simulink model "simula_q10"  (R2018a)
settings: Solver=VariableStepAuto  StartTime=0.0  StopTime=40  RelTol=1e-3
libraries: simulink_extras x9, simulink x6
settings Model: Creator=55479  LastModifiedBy=55479

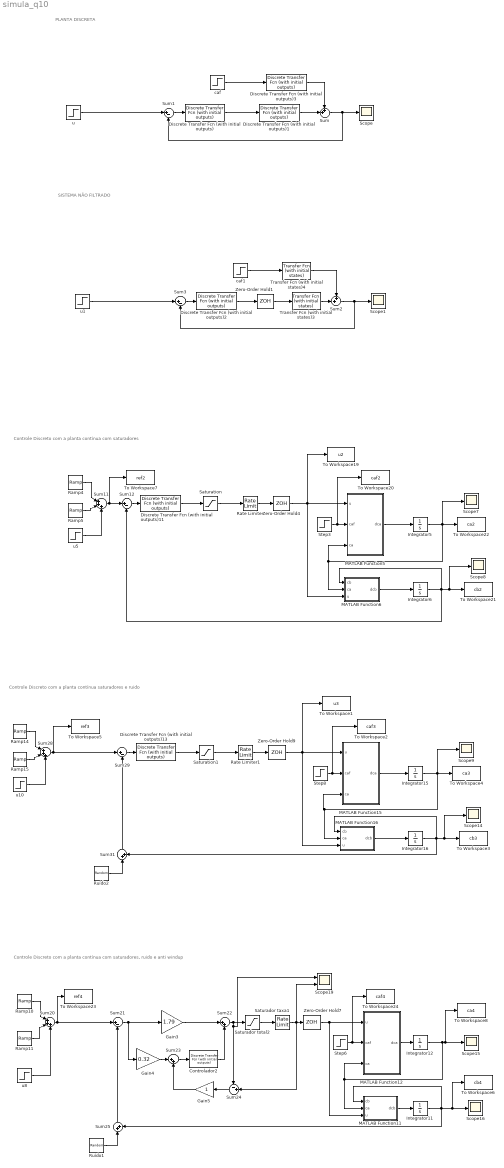
== system simula_q10 ==
  note: SISTEMA NÃO FILTRADO
  note: PLANTA DISCRETA
  note: Controle Discreto com a planta contínua com saturadores
  note: Controle Discreto com a planta contínua saturadores e ruido
  note: Controle Discreto com a planta contínua com saturadores, ruido e anti windup
  Controlador2 : simulink_extras/Additional Discrete/Discrete Transfer Fcn (with initial outputs)  N=[1 0]  D="[1  -1]"  U0=[0]  Y0=0  TS=0.08
      settings: SourceProductName=Simulink  SourceProductBaseCode=SL
  Discrete Transfer Fcn (with initial outputs) : simulink_extras/Additional Discrete/Discrete Transfer Fcn (with initial outputs)  N=[24.2704 -1.7916]  D="[1  -1]"  U0=[1]  Y0=0  TS=0.08
      settings: SourceProductName=Simulink  SourceProductBaseCode=SL
  Discrete Transfer Fcn (with initial outputs)1 : simulink_extras/Additional Discrete/Discrete Transfer Fcn (with initial outputs)  N=[0.07101]  D="[1  -0.8732]"  U0=[1]  Y0=2.345  TS=0.08
      settings: SourceProductName=Simulink  SourceProductBaseCode=SL
  Discrete Transfer Fcn (with initial outputs)11 : simulink_extras/Additional Discrete/Discrete Transfer Fcn (with initial outputs)  N=[2.11 -1.79]  D="[1  -1]"  U0=[0]  Y0=0  TS=0.08
      settings: SourceProductName=Simulink  SourceProductBaseCode=SL
  Discrete Transfer Fcn (with initial outputs)13 : simulink_extras/Additional Discrete/Discrete Transfer Fcn (with initial outputs)  N=[2.11 -1.79]  D="[1  -1]"  U0=[0]  Y0=0  TS=0.08
      settings: SourceProductName=Simulink  SourceProductBaseCode=SL
  Discrete Transfer Fcn (with initial outputs)2 : simulink_extras/Additional Discrete/Discrete Transfer Fcn (with initial outputs)  N=[4.2253 -3.585]  D="[1  -1]"  U0=[0]  Y0=0  TS=0.08
      settings: SourceProductName=Simulink  SourceProductBaseCode=SL
  Discrete Transfer Fcn (with initial outputs)3 : simulink_extras/Additional Discrete/Discrete Transfer Fcn (with initial outputs)  N=[0.05706]  D=[1 -0.8732]  U0=[0]  Y0=0  TS=0.08
      settings: SourceProductName=Simulink  SourceProductBaseCode=SL
  Gain3 : Gain  Gain=1.79
  Gain4 : Gain  Gain=0.32
  Gain5 : Gain
  Integrator{5..6,11..12,15..16} (6 alike) : Integrator
  MATLAB Function11 : MATLAB Function  TreatAsAtomicUnit=on
  MATLAB Function12 : MATLAB Function  TreatAsAtomicUnit=on
  MATLAB Function15 : MATLAB Function  TreatAsAtomicUnit=on
  MATLAB Function16 : MATLAB Function  TreatAsAtomicUnit=on
  MATLAB Function5 : MATLAB Function  TreatAsAtomicUnit=on
  MATLAB Function6 : MATLAB Function  TreatAsAtomicUnit=on
  Ramp10 : simulink/Sources/Ramp  slope=2.345/10  start=0  InitialOutput=0
  Ramp11 : simulink/Sources/Ramp  slope=-2.345/10  start=10  InitialOutput=0
  Ramp14 : simulink/Sources/Ramp  slope=2.345/10  start=0  InitialOutput=0
  Ramp15 : simulink/Sources/Ramp  slope=-2.345/10  start=10  InitialOutput=0
  Ramp4 : simulink/Sources/Ramp  slope=2.345/10  start=0  InitialOutput=0
  Ramp5 : simulink/Sources/Ramp  slope=-2.345/10  start=10  InitialOutput=0
  Rate Limiter : RateLimiter  RisingSlewLimit=2  FallingSlewLimit=-2  SampleTimeMode=inherited
  Rate Limiter1 : RateLimiter  RisingSlewLimit=2  FallingSlewLimit=-2  SampleTimeMode=inherited
  Ruído1 : RandomNumber  Variance=0.001  SampleTime=0.001
  Ruído2 : RandomNumber  Variance=0.001  SampleTime=0.001
  Saturador taxa1 : RateLimiter  RisingSlewLimit=2  FallingSlewLimit=-2  SampleTimeMode=inherited
  Saturador total2 : Saturate  UpperLimit=10  LowerLimit=0
  Saturation : Saturate  UpperLimit=10  LowerLimit=0
  Saturation1 : Saturate  UpperLimit=10  LowerLimit=0
  Scope{,1,7..9,14..16} (8 alike) : Scope
  Scope19 : Scope  NumInputPorts=2
  Step3 : Step  Time=30  Before=5.1  After=5.3  SampleTime=0
  Step6 : Step  Time=30  Before=5.1  After=5.4  SampleTime=0
  Step8 : Step  Time=30  Before=5.1  After=5.4  SampleTime=0
  Sum : Sum  Inputs=++|
  Sum{1,3,12,21,29} (5 alike) : Sum  Inputs=|+-
  Sum11 : Sum  Inputs=|+++
  Sum2 : Sum  Inputs=++|
  Sum20 : Sum  Inputs=|+++
  Sum{22..23,25,31} (4 alike) : Sum  Inputs=|++
  Sum24 : Sum  Inputs=-+|
  Sum28 : Sum  Inputs=|+++
  To Workspace1 : ToWorkspace  VariableName=u3  SaveFormat=Timeseries  SampleTime=-1
  To Workspace19 : ToWorkspace  VariableName=u2  SaveFormat=Timeseries  SampleTime=-1
  To Workspace2 : ToWorkspace  VariableName=caf3  SaveFormat=Timeseries  SampleTime=-1
  To Workspace20 : ToWorkspace  VariableName=caf2  SaveFormat=Timeseries  SampleTime=-1
  To Workspace21 : ToWorkspace  VariableName=cb2  SaveFormat=Timeseries  SampleTime=-1
  To Workspace22 : ToWorkspace  VariableName=ca2  SaveFormat=Timeseries  SampleTime=-1
  To Workspace23 : ToWorkspace  VariableName=ref4  SaveFormat=Timeseries  SampleTime=-1
  To Workspace24 : ToWorkspace  VariableName=caf4  SaveFormat=Timeseries  SampleTime=-1
  To Workspace3 : ToWorkspace  VariableName=cb3  SaveFormat=Timeseries  SampleTime=-1
  To Workspace4 : ToWorkspace  VariableName=ca3  SaveFormat=Timeseries  SampleTime=-1
  To Workspace5 : ToWorkspace  VariableName=ref3  SaveFormat=Timeseries  SampleTime=-1
  To Workspace6 : ToWorkspace  VariableName=cb4  SaveFormat=Timeseries  SampleTime=-1
  To Workspace7 : ToWorkspace  VariableName=ref2  SaveFormat=Timeseries  SampleTime=-1
  To Workspace8 : ToWorkspace  VariableName=ca4  SaveFormat=Timeseries  SampleTime=-1
  Transfer Fcn (with initial states)3 : simulink_extras/Additional Linear/Transfer Fcn (with initial states)  N=[0.56]  D=[0.59 1]  X0=0
  Transfer Fcn (with initial states)4 : simulink_extras/Additional Linear/Transfer Fcn (with initial states)  N=[0.45]  D=[0.59 1]  X0=0
  Zero-Order Hold{1,4,7,9} (4 alike) : ZeroOrderHold  SampleTime=0.08
  caf : Step  Time=10  Before=5.1  After=5.1  SampleTime=0
  caf1 : Step  Time=10  Before=5.1  After=5.1  SampleTime=0
  u : Step  Time=10  Before=2.345  After=2.545  SampleTime=0
  u1 : Step  Time=40  Before=2.345  After=2.545  SampleTime=0.08
  u10 : Step  Time=20  After=0.3  SampleTime=0
  u5 : Step  Time=20  After=0.2  SampleTime=0
  u8 : Step  Time=20  After=0.3  SampleTime=0
  wires:
  Sum/1 -> Sum1/2, Scope/1
  Sum1/1 -> Discrete Transfer Fcn (with initial outputs)/1
  caf/1 -> Discrete Transfer Fcn (with initial outputs)3/1
  u/1 -> Sum1/1
  Zero-Order Hold1/1 -> Transfer Fcn (with initial states)3/1
  Transfer Fcn (with initial states)3/1 -> Sum2/2
  Sum3/1 -> Discrete Transfer Fcn (with initial outputs)2/1
  u1/1 -> Sum3/1
  Sum2/1 -> Scope1/1, Sum3/2
  Transfer Fcn (with initial states)4/1 -> Sum2/1
  Discrete Transfer Fcn (with initial outputs)2/1 -> Zero-Order Hold1/1
  caf1/1 -> Transfer Fcn (with initial states)4/1
  Discrete Transfer Fcn (with initial outputs)3/1 -> Sum/1
  Discrete Transfer Fcn (with initial outputs)1/1 -> Sum/2
  Discrete Transfer Fcn (with initial outputs)/1 -> Discrete Transfer Fcn (with initial outputs)1/1
  Ramp5/1 -> Sum11/2
  MATLAB Function5/1(dca) -> Integrator5/1
  u5/1 -> Sum11/3
  MATLAB Function6/1(dcb) -> Integrator6/1
  Ramp4/1 -> Sum11/1
  Integrator6/1 -> Sum12/2, MATLAB Function6/1(cb), Scope8/1, To Workspace21/1
  Step3/1 -> To Workspace20/1, MATLAB Function5/2(caf)
  Sum12/1 -> Discrete Transfer Fcn (with initial outputs)11/1
  Zero-Order Hold4/1 -> To Workspace19/1, MATLAB Function6/3(u), MATLAB Function5/1(u)
  Integrator5/1 -> To Workspace22/1, Scope7/1, MATLAB Function6/2(ca), MATLAB Function5/3(ca)
  Saturation/1 -> Rate Limiter/1
  Rate Limiter/1 -> Zero-Order Hold4/1
  Discrete Transfer Fcn (with initial outputs)11/1 -> Saturation/1
  Sum11/1 -> Sum12/1, To Workspace7/1
  Integrator15/1 -> To Workspace4/1, Scope9/1, MATLAB Function16/2(ca), MATLAB Function15/3(ca)
  Sum28/1 -> Sum29/1, To Workspace5/1
  Sum29/1 -> Discrete Transfer Fcn (with initial outputs)13/1
  MATLAB Function16/1(dcb) -> Integrator16/1
  MATLAB Function15/1(dca) -> Integrator15/1
  Zero-Order Hold9/1 -> To Workspace1/1, MATLAB Function16/3(u), MATLAB Function15/1(u)
  Discrete Transfer Fcn (with initial outputs)13/1 -> Saturation1/1
  Saturation1/1 -> Rate Limiter1/1
  Ramp14/1 -> Sum28/1
  Rate Limiter1/1 -> Zero-Order Hold9/1
  Step8/1 -> To Workspace2/1, MATLAB Function15/2(caf)
  Ramp15/1 -> Sum28/2
  u10/1 -> Sum28/3
  Integrator16/1 -> Sum31/2, MATLAB Function16/1(cb), Scope14/1, To Workspace3/1
  Saturador taxa1/1 -> Sum24/2, Scope19/2, Zero-Order Hold7/1
  MATLAB Function12/1(dca) -> Integrator12/1
  Saturador total2/1 -> Saturador taxa1/1
  Sum21/1 -> Gain4/1, Gain3/1
  Integrator11/1 -> Sum25/2, MATLAB Function11/1(cb), To Workspace6/1, Scope16/1
  Zero-Order Hold7/1 -> MATLAB Function11/3(u), MATLAB Function12/1(u)
  Sum24/1 -> Gain5/1
  Gain4/1 -> Sum23/1
  Integrator12/1 -> To Workspace8/1, Scope15/1, MATLAB Function12/3(ca), MATLAB Function11/2(ca)
  Gain3/1 -> Sum22/1
  Gain5/1 -> Sum23/2
  Controlador2/1 -> Sum22/2
  Ramp11/1 -> Sum20/2
  Sum23/1 -> Controlador2/1
  u8/1 -> Sum20/3
  MATLAB Function11/1(dcb) -> Integrator11/1
  Sum22/1 -> Scope19/1, Sum24/1, Saturador total2/1
  Ramp10/1 -> Sum20/1
  Sum20/1 -> Sum21/1, To Workspace23/1
  Step6/1 -> To Workspace24/1, MATLAB Function12/2(caf)
  Sum25/1 -> Sum21/2
  Ruído1/1 -> Sum25/1
  Sum31/1 -> Sum29/2
  Ruído2/1 -> Sum31/1

== matlab function simula_q10/MATLAB Function5 ==
  data: u input; dca output; caf input; ca input
function dca = fcn(u,caf,ca)
k1=6.01;
k2=0.8433;
k3=0.1123;
dca = (-k1*ca)-(k3*ca^2)+((caf-ca)*u);

== matlab function simula_q10/MATLAB Function6 ==
  data: cb input; ca input; u input; dcb output
function dcb = fcn(cb,ca,u)
k1=6.01;
k2=0.8433;
k3=0.1123;
dcb = k1*ca-(k2*cb)-(cb*u);

== matlab function simula_q10/MATLAB Function11 ==
  data: cb input; ca input; u input; dcb output
function dcb = fcn(cb,ca,u)
k1=6.01;
k2=0.8433;
k3=0.1123;
dcb = k1*ca-(k2*cb)-(cb*u);

== matlab function simula_q10/MATLAB Function12 ==
  data: u input; dca output; caf input; ca input
function dca = fcn(u,caf,ca)
k1=6.01;
k2=0.8433;
k3=0.1123;
dca = (-k1*ca)-(k3*ca^2)+((caf-ca)*u);

== matlab function simula_q10/MATLAB Function15 ==
  data: u input; dca output; caf input; ca input
function dca = fcn(u,caf,ca)
k1=6.01;
k2=0.8433;
k3=0.1123;
dca = (-k1*ca)-(k3*ca^2)+((caf-ca)*u);

== matlab function simula_q10/MATLAB Function16 ==
  data: cb input; ca input; u input; dcb output
function dcb = fcn(cb,ca,u)
k1=6.01;
k2=0.8433;
k3=0.1123;
dcb = k1*ca-(k2*cb)-(cb*u);
